simulink model "IFinc"  (R2021a)
settings: Solver=ode4  StartTime=0.0  StopTime=60000.0  FixedStep=1  RelTol=1e-3
undefined symbols (not defined in the file or in its folder): Ca, Cb, Fa, K, Kd_cap, Kp_cap, Ku_cap, kw, sel, Ti, Tt, uep, V
libraries: eeGeneralControl x1, fuzblock x1
settings Model: Creator=svorc  LastModifiedBy=svorc

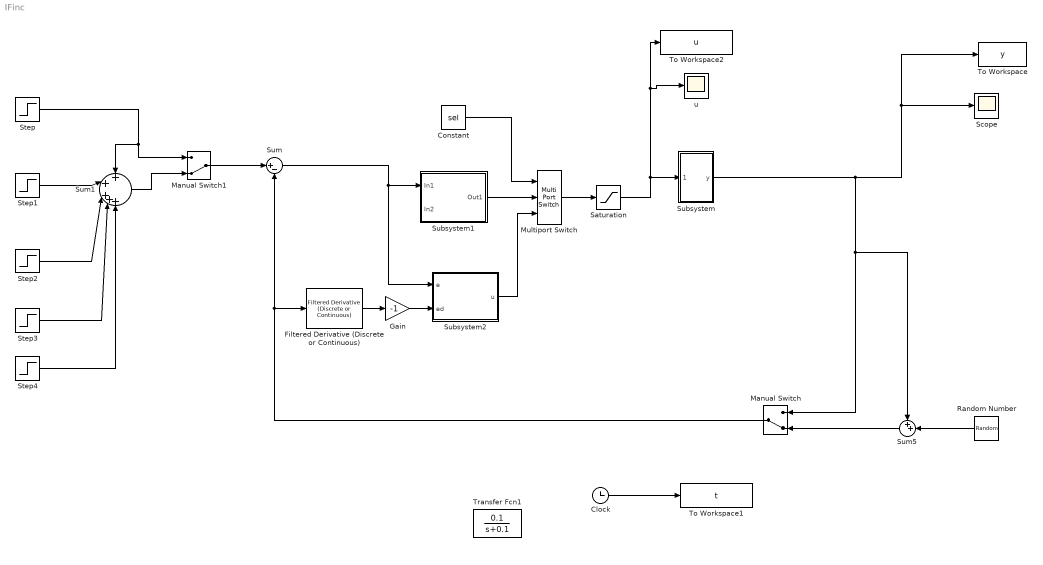
== system IFinc ==
  Clock : Clock
  Constant : Constant  Value=sel
  Filtered Derivative (Discrete or Continuous) : eeGeneralControl/Filtered Derivative (Discrete or Continuous)  K=1  T=1  B=inf  A=-inf  minRatio=10  init_option=Inherited from block input  x0=0  Ts=-1
      settings: SourceProductBaseCode=PS
  Gain : Gain  Gain=-1
  Manual Switch : ManualSwitch  CurrentSetting=0
  Manual Switch1 : ManualSwitch  CurrentSetting=0
  Multiport Switch : MultiPortSwitch  Inputs=2
  Random Number : RandomNumber  Variance=0.1225  SampleTime=1
  Saturation : Saturate  UpperLimit=10*Fa  LowerLimit=0
  Scope : Scope
  Step : Step  Time=0  After=7  SampleTime=0
  Step1 : Step  Time=10000  After=-0.5  SampleTime=0
  Step2 : Step  Time=20000  After=0.5  SampleTime=0
  Step3 : Step  Time=30000  After=0.5  SampleTime=0
  Step4 : Step  Time=40000  After=-0.5  SampleTime=0
  Subsystem : Subsystem
  Subsystem1 : Subsystem
  Subsystem2 : Subsystem
  Sum : Sum  Inputs=|+-
  Sum1 : Sum  Inputs=+|+|+++
  Sum5 : Sum  Inputs=++|
  To Workspace : ToWorkspace  VariableName=y  SampleTime=-1
  To Workspace1 : ToWorkspace  VariableName=t  SampleTime=-1
  To Workspace2 : ToWorkspace  VariableName=u  SampleTime=-1
  Transfer Fcn1 : TransferFcn  Numerator=[0.1]  Denominator=[1 0.1]
  u : Scope
  wires:
  Sum5/1 -> Manual Switch/2
  Clock/1 -> To Workspace1/1
  Step4/1 -> Sum1/5
  Sum1/1 -> Manual Switch1/2
  Step1/1 -> Sum1/2
  Step/1 -> Manual Switch1/1, Sum1/1
  Step3/1 -> Sum1/4
  Random Number/1 -> Sum5/2
  Subsystem/1(y) -> Manual Switch/1, Sum5/1, Scope/1, To Workspace/1
  Manual Switch1/1 -> Sum/1
  Step2/1 -> Sum1/3
  Sum/1 -> Subsystem2/1(e), Subsystem1/1(In1)
  Saturation/1 -> u/1, To Workspace2/1, Subsystem/1(Input)
  Gain/1 -> Subsystem2/2(ed)
  Filtered Derivative (Discrete or Continuous)/1 -> Gain/1
  Manual Switch/1 -> Filtered Derivative (Discrete or Continuous)/1, Sum/2
  Multiport Switch/1 -> Saturation/1
  Subsystem1/1(Out1) -> Multiport Switch/2
  Subsystem2/1(u) -> Multiport Switch/3
  Constant/1 -> Multiport Switch/1

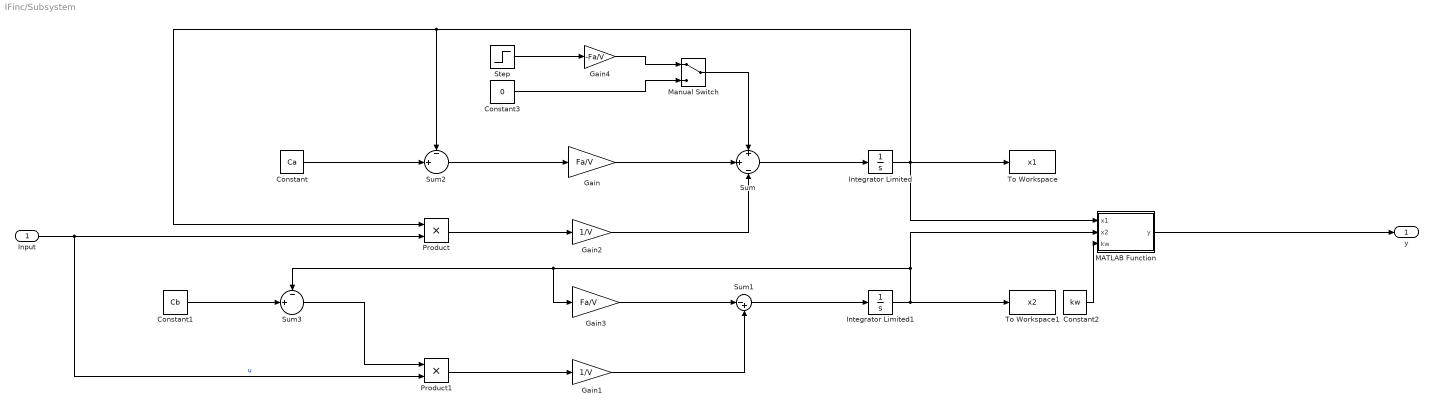
== system IFinc/Subsystem ==
  Input : Inport
  Constant : Constant  Value=Ca
  Constant1 : Constant  Value=Cb
  Constant2 : Constant  Value=kw
  Constant3 : Constant  Value=0
  Gain : Gain  Gain=Fa/V
  Gain1 : Gain  Gain=1/V
  Gain2 : Gain  Gain=1/V
  Gain3 : Gain  Gain=Fa/V
  Gain4 : Gain  Gain=-Fa/V
  Integrator Limited : Integrator  LimitOutput=on  UpperSaturationLimit=Ca  LowerSaturationLimit=0
  Integrator Limited1 : Integrator  LimitOutput=on  UpperSaturationLimit=Cb  LowerSaturationLimit=0
  MATLAB Function : MATLAB Function  TreatAsAtomicUnit=on
  Manual Switch : ManualSwitch
  Product : Product
  Product1 : Product
  Step : Step  Time=50000  After=0.5*Ca  SampleTime=0
  Sum : Sum  Inputs=+|+|-
  Sum1 : Sum  Inputs=|-+
  Sum2 : Sum  Inputs=-|+||
  Sum3 : Sum  Inputs=-|+||
  To Workspace : ToWorkspace  VariableName=x1  SampleTime=-1
  To Workspace1 : ToWorkspace  VariableName=x2  SampleTime=-1
  y : Outport
  wires:
  Sum3/1 -> Product1/1
  Sum/1 -> Integrator Limited/1
  Gain/1 -> Sum/2
  Input/1 -> Product/2, Product1/2  "u"
  Gain3/1 -> Sum1/1
  Integrator Limited1/1 -> MATLAB Function/2(x2), Gain3/1, Sum3/1, To Workspace1/1
  Integrator Limited/1 -> To Workspace/1, MATLAB Function/1(x1), Sum2/1, Product/1
  Constant1/1 -> Sum3/2
  Sum1/1 -> Integrator Limited1/1
  Product1/1 -> Gain1/1
  Constant/1 -> Sum2/2
  MATLAB Function/1(y) -> y/1
  Gain1/1 -> Sum1/2
  Product/1 -> Gain2/1
  Sum2/1 -> Gain/1
  Constant2/1 -> MATLAB Function/3(kw)
  Gain2/1 -> Sum/3
  Step/1 -> Gain4/1
  Manual Switch/1 -> Sum/1
  Gain4/1 -> Manual Switch/1
  Constant3/1 -> Manual Switch/2

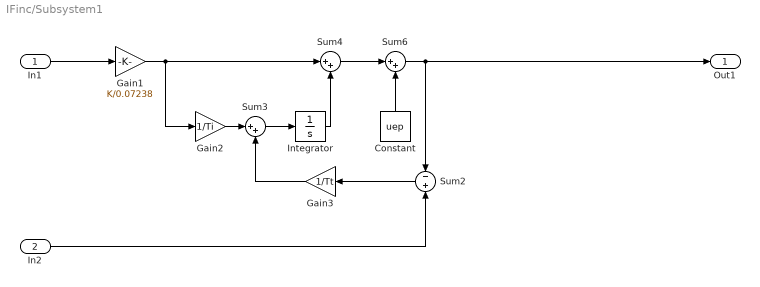
== system IFinc/Subsystem1 ==
  In1 : Inport
  In2 : Inport  Port=2
  Constant : Constant  Value=uep
  Gain1 : Gain  Gain=K/0.07238
  Gain2 : Gain  Gain=1/Ti
  Gain3 : Gain  Gain=1/Tt
  Integrator : Integrator
  Sum2 : Sum  Inputs=-|+
  Sum3 : Sum  Inputs=|++
  Sum4 : Sum  Inputs=|++
  Sum6 : Sum  Inputs=|++
  Out1 : Outport
  wires:
  Sum4/1 -> Sum6/1
  Constant/1 -> Sum6/2
  Sum2/1 -> Gain3/1
  Integrator/1 -> Sum4/2
  Gain1/1 -> Gain2/1, Sum4/1
  Gain3/1 -> Sum3/2
  Sum6/1 -> Out1/1, Sum2/1
  In2/1 -> Sum2/2
  Gain2/1 -> Sum3/1
  Sum3/1 -> Integrator/1
  In1/1 -> Gain1/1

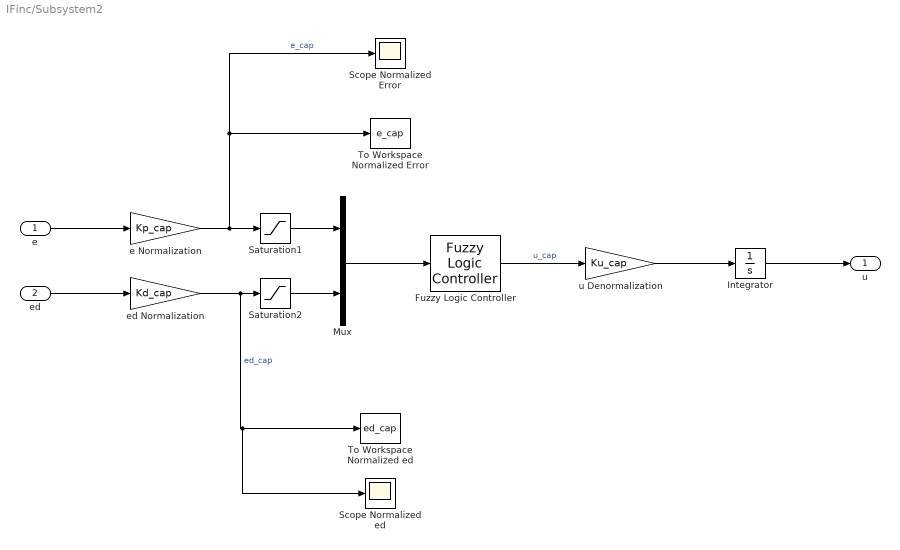
== system IFinc/Subsystem2 ==
  e : Inport
  ed : Inport  Port=2
  Fuzzy Logic Controller : fuzblock/Fuzzy Logic  Controller  FIS='lin_fpd_blaga.fis'  OutputSampleNumber=101  DataType=double  FuzzifiedInputs=off  RuleFiringStrengths=off  RuleOutputs=off  AggregatedOutputs=off  SimulateUsing=Interpreted execution  OutOfRangeInputValueMessage=warning  NoRuleFiredMessage=warning  EmptyOutputFuzzySetMessage=warning
  Integrator : Integrator
  Mux : Mux  Inputs=2
  Saturation1 : Saturate  UpperLimit=1  LowerLimit=-1
  Saturation2 : Saturate  UpperLimit=1  LowerLimit=-1
  Scope Normalized Error : Scope
  Scope Normalized ed : Scope
  To Workspace Normalized Error : ToWorkspace  VariableName=e_cap  SampleTime=-1
  To Workspace Normalized ed : ToWorkspace  VariableName=ed_cap  SampleTime=-1
  e Normalization : Gain  Gain=Kp_cap  SaturateOnIntegerOverflow=on  OutDataTypeStr=Inherit: Same as input  ParamDataTypeStr=Inherit: Same as input
  ed Normalization : Gain  Gain=Kd_cap  SaturateOnIntegerOverflow=on  OutDataTypeStr=Inherit: Same as input  ParamDataTypeStr=Inherit: Same as input
  u Denormalization : Gain  Gain=Ku_cap  SaturateOnIntegerOverflow=on  OutDataTypeStr=Inherit: Same as input  ParamDataTypeStr=Inherit: Same as input
  u : Outport
  wires:
  Mux/1 -> Fuzzy Logic Controller/1
  Saturation2/1 -> Mux/2
  Saturation1/1 -> Mux/1
  e/1 -> e Normalization/1
  ed/1 -> ed Normalization/1
  u Denormalization/1 -> Integrator/1
  Integrator/1 -> u/1
  e Normalization/1 -> Scope Normalized Error/1, To Workspace Normalized Error/1, Saturation1/1  "e_cap"
  Fuzzy Logic Controller/1 -> u Denormalization/1  "u_cap"
  ed Normalization/1 -> To Workspace Normalized ed/1, Scope Normalized ed/1, Saturation2/1  "ed_cap"

== matlab function IFinc/Subsystem/MATLAB Function ==
  data: x1 input; y output; x2 input; kw input
function y = fcn(x1, x2, kw)

y = -log10(sqrt((x2-x1)^2 / 4 + kw) - (x2 - x1) / 2);
